simulink model "FlowControllerPrototype"  (R2021a)
settings: Solver=VariableStepAuto  StartTime=0.0  StopTime=10.0  RelTol=1e-3
settings Model: Creator=phill  LastModifiedBy=phill

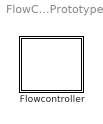
== system FlowControllerPrototype ==
  Flowcontroller : Stateflow chart  TreatAsAtomicUnit=on

== stateflow chart FlowControllerPrototype/Flowcontroller ==
  state Disabled
    flow=0
  state Enabled
    flow=1
  (default) -> Disabled
  Disabled -> Enabled
  Enabled -> Disabled
